simulink model "Servo_Benchmark"  (R2022b)
settings: Solver=ode23t  StartTime=0.0  StopTime=20  RelTol=1e-3
undefined symbols (not defined in the file or in its folder): LF
libraries: instrumentseriallib x3, simulink x2, svdutilitieslib x1
settings Model: PacingRate=10  Creator=gotta  LastModifiedBy=gotta
settings ExplorerConfigSet: InternalSimMechanicsExplorerSettings="<ExplorerConfiguration><canonicalview>default</canonicalview><AnimationSetting><BasePlaybackSpeed>1.0</BasePlaybackSpeed><PlaybackSpeedFactor>1.0</PlaybackSpeedFactor></AnimationSetting><TilePanel><TileInfo><Tiles Columns=\"2\" Count=\"3\" Rows=\"2\"><Column Weight=\"0.4994\"/><Column Weight=\"0.5006\"/><Row Weight=\"0.4993\"/><Row Weight=\"0.5007\"/><Tile Height=\"2\" Width=\"1\" X=\"0\" Y=\"0\"/><Tile Height=\"1\" Width=\"1\" X=\"1\" Y=\"0\"/><Tile Height=\"1\" Width=\"1\" X=\"1\" Y=\"1\"/></Tiles></TileInfo><SceneInfo><SceneViewer><BGColor><R>0.60000002384185791</R><G>0.60000002384185791</G><B>0.60000002384185791</B></BGColor><Camera><DoPerspective>off</DoPerspective><Position><X>0.130605904800483619</X><Y>-1.03965353021318974</Y><Z>0.165975841105155203</Z></Position><Center><X>0.130605904800483619</X><Y>-0.039653530213189736</Y><Z>0.165975841105155203</Z></Center><Up><X>0</X><Y>-0</Y><Z>1</Z></Up><ViewLimDist>1</ViewLimDist><YLim>0.285256663070233507</YLim><XLim>0.289401740076538072</XLim></Camera></SceneViewer><SceneViewer><BGColor><R>0.60000002384185791</R><G>0.60000002384185791</G><B>0.60000002384185791</B></BGColor><Camera><DoPerspective>off</DoPerspective><Position><X>0.102066420747171926</X><Y>-0.000570082663057591005</Y><Z>1.10062331896404597</Z></Position><Center><X>0.102066420747171926</X><Y>-0.000570082663057591005</Y><Z>0.100623318964045971</Z></Center><Up><X>0</X><Y>1</Y><Z>-0</Z></Up><ViewLimDist>1</ViewLimDist><YLim>0.171233923815175632</YLim><XLim>0.352540431384185116</XLim></Camera></SceneViewer><SceneViewer><BGColor><R>0.60000002384185791</R><G>0.60000002384185791</G><B>0.60000002384185791</B></BGColor><Camera><DoPerspective>off</DoPerspective><Position><X>1.08629246460336626</X><Y>-0.00159593778916227759</Y><Z>0.183546684797173593</Z></Position><Center><X>0.086292464603366259</X><Y>-0.00159593778916227759</Y><Z>0.183546684797173593</Z></Center><Up><X>-0</X><Y>0</Y><Z>1</Z></Up><ViewLimDist>1</ViewLimDist><YLim>0.219665879586588786</YLim><XLim>0.452253281501800386</XLim></Camera></SceneViewer></SceneInfo></TilePanel><MechEditorPanel><Cameras/><GfxPanelCameraMap/><VideoCreator><PlaybackSpeedRatio>1.0</PlaybackSpeedRatio><FrameRate>30</FrameRate><VideoFormat>Motion JPEG AVI</VideoFormat><FrameSize>auto</FrameSize></VideoCreator></MechEditorPanel></ExplorerConfiguration>"

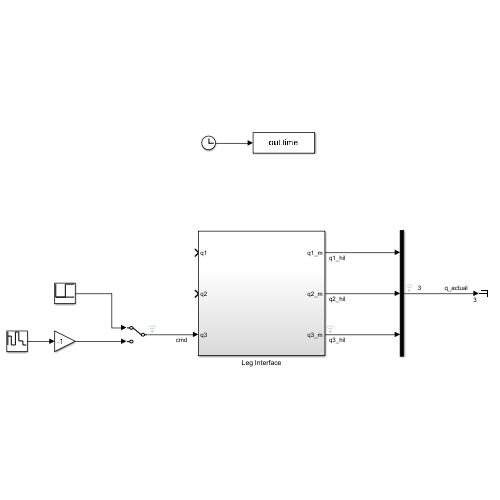
[thumbnail: Simulink's stored preview of the top-level diagram]
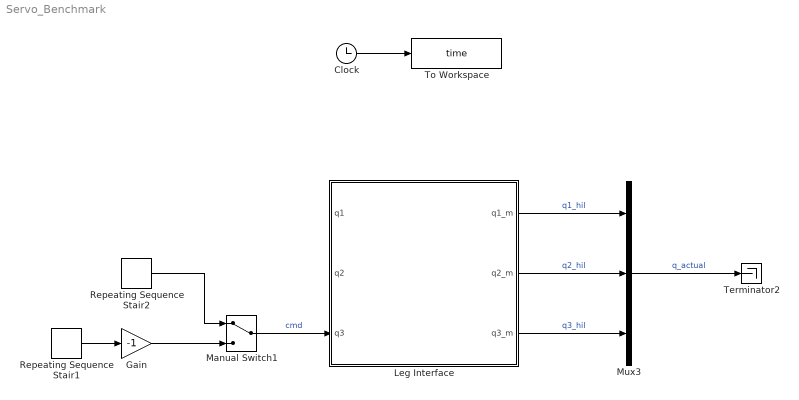
== system Servo_Benchmark ==
  Clock : Clock
  Gain : Gain  Gain=-1
  Leg Interface : Subsystem
  Manual Switch1 : ManualSwitch
  Mux3 : Mux  Inputs=3
  Repeating Sequence Stair1 : simulink/Sources/Repeating Sequence Stair  OutValues=[-2000:1:2000]  tsamp=1e-1  OutMin=[]  OutMax=[]  OutDataTypeStr=double  OutputDataTypeScalingMode=double  OutDataType=fixdt(0,8)  ConRadixGroup=Best Precision: Vector-wise  OutScaling=2^-12
  Repeating Sequence Stair2 : simulink/Sources/Repeating Sequence Stair  OutValues=[0, 90*2048/180]  tsamp=2  OutMin=[]  OutMax=[]  OutDataTypeStr=double  OutputDataTypeScalingMode=double  OutDataType=fixdt(0,8)  ConRadixGroup=Best Precision: Vector-wise  OutScaling=2^-12
  Terminator2 : Terminator
  To Workspace : ToWorkspace  VariableName=time  SampleTime=1e-4
      settings: Save2DSignal=2-D array (concatenate along first dimension)
  wires:
  Leg Interface/3(q3_m) -> Mux3/3  "q3_hil"
  Leg Interface/2(q2_m) -> Mux3/2  "q2_hil"
  Leg Interface/1(q1_m) -> Mux3/1  "q1_hil"
  Repeating Sequence Stair2/1 -> Manual Switch1/1
  Mux3/1 -> Terminator2/1  "q_actual"
  Repeating Sequence Stair1/1 -> Gain/1
  Clock/1 -> To Workspace/1
  Manual Switch1/1 -> Leg Interface/3(q3)  "cmd"
  Gain/1 -> Manual Switch1/2

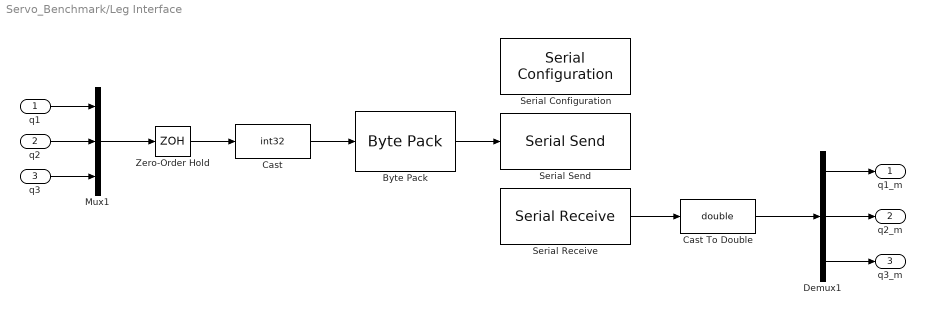
== system Servo_Benchmark/Leg Interface ==
  q1 : Inport
  q2 : Inport  Port=2
  q3 : Inport  Port=3
  Byte Pack : svdutilitieslib/Byte Pack  maskPackedDataType=uint8  datatypes={'int32'}  byteAlign=1  blockPlatform=arduinoert
  Cast : DataTypeConversion  OutDataTypeStr=int32  SaturateOnIntegerOverflow=off  RndMeth=Floor
  Cast To Double : DataTypeConversion  OutDataTypeStr=double  SaturateOnIntegerOverflow=off  RndMeth=Floor
  Demux1 : Demux  Outputs=3
  Mux1 : Mux  Inputs=3
  Serial Configuration : instrumentseriallib/Serial Configuration  Priority=-200000  PortSel=COM6  Port=COM6  ComPort=COM6  BaudRate=115200  DataBits=8  Parity=none  StopBits=1  ByteOrder=little-endian  FlowControl=none  Timeout=10  SimulateUsing=Interpreted execution  BlockInModel=on  aMode=1
  Serial Receive : instrumentseriallib/Serial Receive  Priority=1  PortSel=COM6  Port=COM6  ComPort=COM6  DataType=int32  SaveDataType=uint8  ToggleHeader=on  Header='A'  ToggleTerminator=on  Terminator=LF ('\n')  CustomTerminator=[]  InputFormat=Column major  ToggleDataSize=on  DataSize=[1 3]  EnableBlockingMode=on  ActionDataUnavailable=Output last received value  ActionWhenDataUnavailable=Output last received value  CustomValue=0  SampleTime=1e-2  SimulateUsing=Interpreted execution  BlockInModel=on  aMode=1
  Serial Send : instrumentseriallib/Serial Send  Priority=1  PortSel=COM6  Port=COM6  ComPort=COM6  Header=[]  Terminator=<none>  CustomTerminator=[]  EnableBlockingMode=on  SimulateUsing=Interpreted execution  BlockInModel=on  aMode=1
  Zero-Order Hold : ZeroOrderHold  SampleTime=1e-2
  q1_m : Outport
  q2_m : Outport  Port=2
  q3_m : Outport  Port=3
  wires:
  Cast/1 -> Byte Pack/1
  Serial Receive/1 -> Cast To Double/1
  Demux1/2 -> q2_m/1
  Demux1/1 -> q1_m/1
  q1/1 -> Mux1/1
  q2/1 -> Mux1/2
  Cast To Double/1 -> Demux1/1
  Mux1/1 -> Zero-Order Hold/1
  Byte Pack/1 -> Serial Send/1
  Zero-Order Hold/1 -> Cast/1
  q3/1 -> Mux1/3
  Demux1/3 -> q3_m/1
